simulink model "dc_motor"  (R2021b)
settings: Solver=VariableStepAuto  StartTime=0.0  StopTime=10.0  MaxStep=15e-3  RelTol=1e-3
undefined symbols (not defined in the file): b, J, k_e, k_p, k_t, L_a, R_a, T_0, tau, V_nom
libraries: simulink x1
settings Model: Creator=Oleg  LastModifiedBy=Oleg
settings DataIOCC: ReturnWorkspaceOutputsName=SDOSimTest_Log

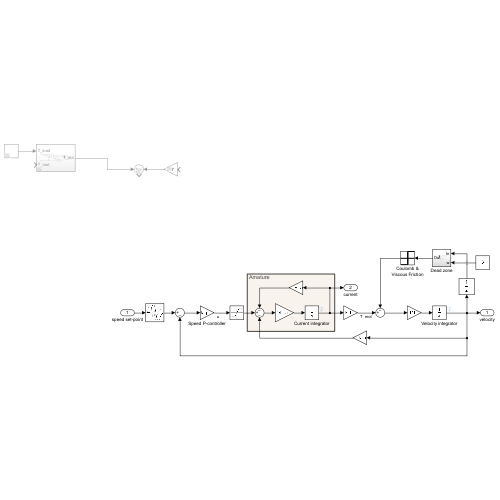
[thumbnail: Simulink's stored preview of the top-level diagram]
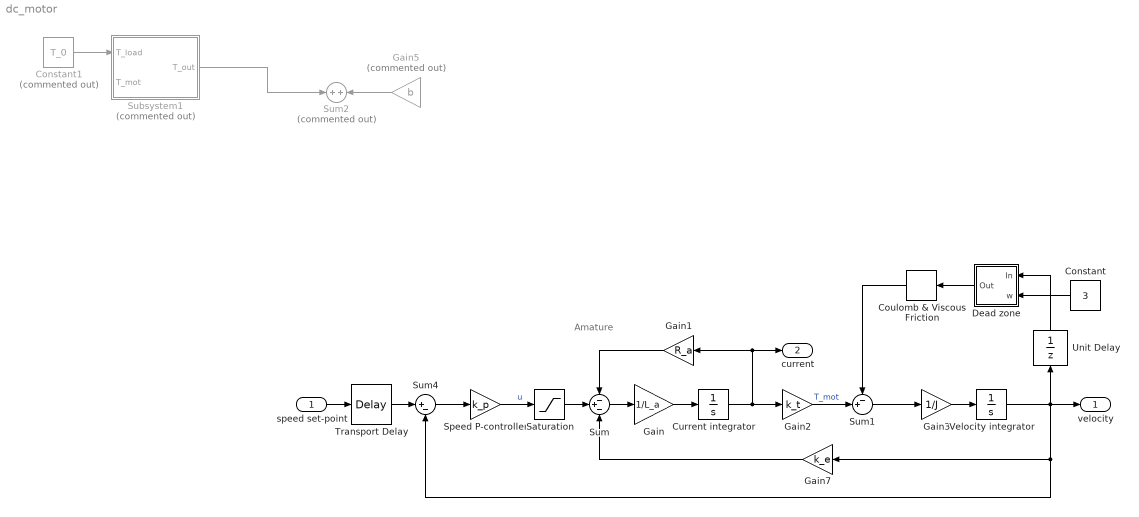
== system dc_motor ==
  note: Amature
  speed set-point : Inport
  Constant : Constant  Value=3
  Constant1 : Constant  Commented=on  Value=T_0
  Coulomb & Viscous Friction : simulink/Discontinuities/Coulomb & Viscous Friction  offset=T_0  gain=b
  Current integrator : Integrator
  Dead zone : Subsystem
  Gain : Gain  Gain=1/L_a
  Gain1 : Gain  Gain=R_a
  Gain2 : Gain  Gain=k_t
  Gain3 : Gain  Gain=1/J
  Gain5 : Gain  Commented=on  Gain=b
  Gain7 : Gain  Gain=k_e
  Saturation : Saturate  UpperLimit=V_nom  LowerLimit=-V_nom
  Speed P-controller : Gain  Gain=k_p
  Subsystem1 : Subsystem  Commented=on
  Sum : Sum  Inputs=-+-
  Sum1 : Sum  Inputs=-+|
  Sum2 : Sum  Commented=on  Inputs=+|+
  Sum4 : Sum  Inputs=|+-
  Transport Delay : TransportDelay  DelayTime=tau
  Unit Delay : UnitDelay  SampleTime=-1  HasFrameUpgradeWarning=on
  Velocity integrator : Integrator
  velocity : Outport
  current : Outport  Port=2
  wires:
  Gain/1 -> Current integrator/1
  Sum/1 -> Gain/1
  Gain1/1 -> Sum/1
  Current integrator/1 -> Gain2/1, current/1, Gain1/1
  Gain2/1 -> Sum1/2  "T_mot"
  Sum1/1 -> Gain3/1
  Gain3/1 -> Velocity integrator/1
  Velocity integrator/1 -> Unit Delay/1, velocity/1, Sum4/2, Gain7/1
  Gain7/1 -> Sum/3
  Sum4/1 -> Speed P-controller/1
  Constant/1 -> Dead zone/2(w)
  Unit Delay/1 -> Dead zone/1(In)
  Gain5/1 -> Sum2/2
  Constant1/1 -> Subsystem1/1(T_load)
  Subsystem1/1(T_out) -> Sum2/1
  Dead zone/1(Out) -> Coulomb & Viscous Friction/1
  Saturation/1 -> Sum/2
  Speed P-controller/1 -> Saturation/1  "u"
  speed set-point/1 -> Transport Delay/1
  Transport Delay/1 -> Sum4/1
  Coulomb & Viscous Friction/1 -> Sum1/1

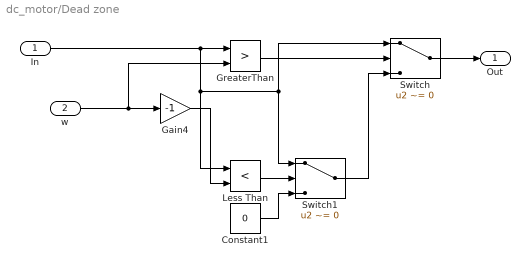
== system dc_motor/Dead zone ==
  In : Inport
  w : Inport  Port=2
  Constant1 : Constant  Value=0
  Gain4 : Gain  Gain=-1
  GreaterThan : RelationalOperator  Operator=>  OutDataTypeStr=boolean  RndMeth=Simplest
  Less Than : RelationalOperator  Operator=<  OutDataTypeStr=boolean  RndMeth=Simplest
  Switch : Switch  Criteria=u2 ~= 0
  Switch1 : Switch  Criteria=u2 ~= 0
  Out : Outport
  wires:
  w/1 -> Gain4/1, GreaterThan/2
  Switch1/1 -> Switch/3
  Gain4/1 -> Less Than/2
  Switch/1 -> Out/1
  Less Than/1 -> Switch1/2
  GreaterThan/1 -> Switch/2
  In/1 -> Switch/1, Switch1/1, Less Than/1, GreaterThan/1
  Constant1/1 -> Switch1/3

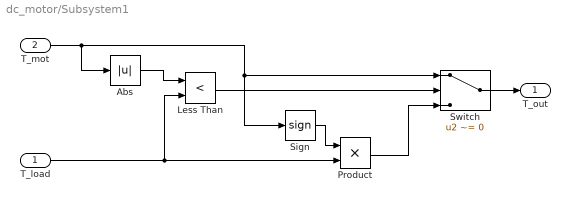
== system dc_motor/Subsystem1 ==
  T_load : Inport
  T_mot : Inport  Port=2
  Abs : Abs
  Less Than : RelationalOperator  Operator=<  OutDataTypeStr=boolean  RndMeth=Simplest
  Product : Product
  Sign : Signum
  Switch : Switch  Criteria=u2 ~= 0
  T_out : Outport
  wires:
  T_load/1 -> Product/2, Less Than/2
  Less Than/1 -> Switch/2
  T_mot/1 -> Sign/1, Switch/1, Abs/1
  Switch/1 -> T_out/1
  Abs/1 -> Less Than/1
  Sign/1 -> Product/1
  Product/1 -> Switch/3
